simulink model "SIQBSC9LI"  (R2016a)
settings: Solver=VariableStepAuto  StartTime=0.0  StopTime=4/50  MaxStep=1e-6  MinStep=1e-7  RelTol=1e-3
libraries: powerlib x27
settings Model: Creator=satheeshwaran  LastModifiedBy=satheeshwaran

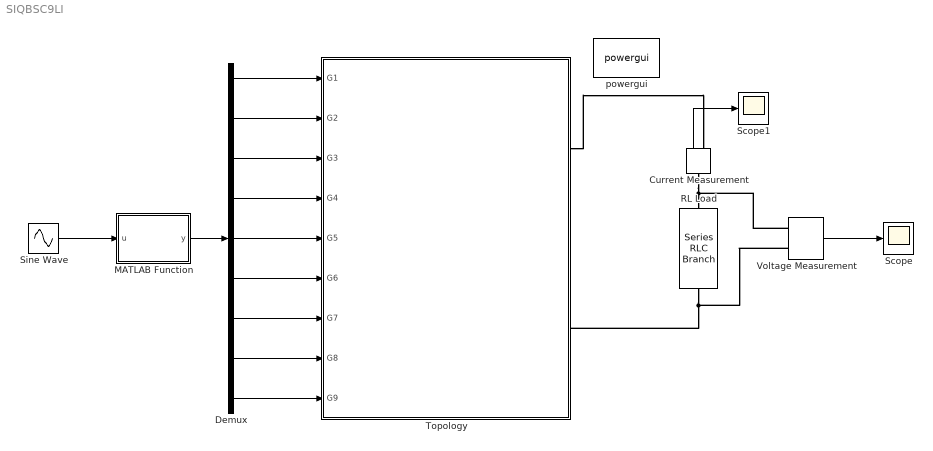
== system SIQBSC9LI ==
  Current Measurement : powerlib/Measurements/Current Measurement  PhasorSimulation=off  OutputType=Complex  PSBequivalent=0
  Demux : Demux  Outputs=9
  MATLAB Function : MATLAB Function  TreatAsAtomicUnit=on
  RL Load : powerlib/Elements/Series RLC Branch  LConnTagsString=__new0  RConnTagsString=__new0  BranchType=RL  Resistance=50  Inductance=0.1  SetiL0=off  InitialCurrent=0  Capacitance=1e-6  Setx0=off  InitialVoltage=0  Measurements=None
  Scope : Scope
  Scope1 : Scope
  Sine Wave : Sin  Amplitude=4  Frequency=2*pi*50  SampleTime=0
  Topology : Subsystem
  Voltage Measurement : powerlib/Measurements/Voltage Measurement  PhasorSimulation=off  OutputType=Complex  PSBequivalent=0
  powergui : powerlib/powergui  Priority=1  SimulationMode=Continuous  SolverType=Tustin/Backward Euler (TBE)  SampleTime=5e-6  frequency=60  SPID=off  DisableSnubberDevices=off  DisableRonSwitches=off  DisableVfSwitches=off  SwTol=0  DisplayEquations=off  Interpol=off  ExternalGateDelay=off  methode=off  Ts=10  FunctionMessages=off  echomessages=off  HookPort=off  EnableUseOfTLC=off  x0status=blocks  frequencyindice=0  Pbase=100e6  ErrMax=1e-4  Iterations=50  UnitsV=kV  UnitsW=MW  buscounter=0  RestoreLinks=warning  ResistiveCurrentMeasurement=off  Frange=[0:2:500]  Ylog=off  Xlog=on  ShowGrid=off  save=off  variable=ZData  structure=load  ZoomFFT=off  StartTime=0.08  cycles=1  DisplayStyle=1  fundamental=50  FreqAxis=off  MaxFrequency=10000  frequencyindicesteady=1  RmsSteady=1  display=off
  wires:
  Voltage Measurement/1 -> Scope/1
  Sine Wave/1 -> MATLAB Function/1(u)
  Demux/1 -> Topology/1(G1)
  Demux/2 -> Topology/2(G2)
  Demux/3 -> Topology/3(G3)
  Demux/4 -> Topology/4(G4)
  Demux/5 -> Topology/5(G5)
  Demux/6 -> Topology/6(G6)
  Demux/7 -> Topology/7(G7)
  Demux/8 -> Topology/8(G8)
  Demux/9 -> Topology/9(G9)
  MATLAB Function/1(y) -> Demux/1
  Current Measurement/1 -> Scope1/1
  connections:
  Voltage Measurement/LConn1 -- Current Measurement/LConn1 -- RL Load/LConn1
  RL Load/RConn1 -- Voltage Measurement/LConn2 -- Topology/RConn2
  Topology/RConn1 -- Current Measurement/RConn1

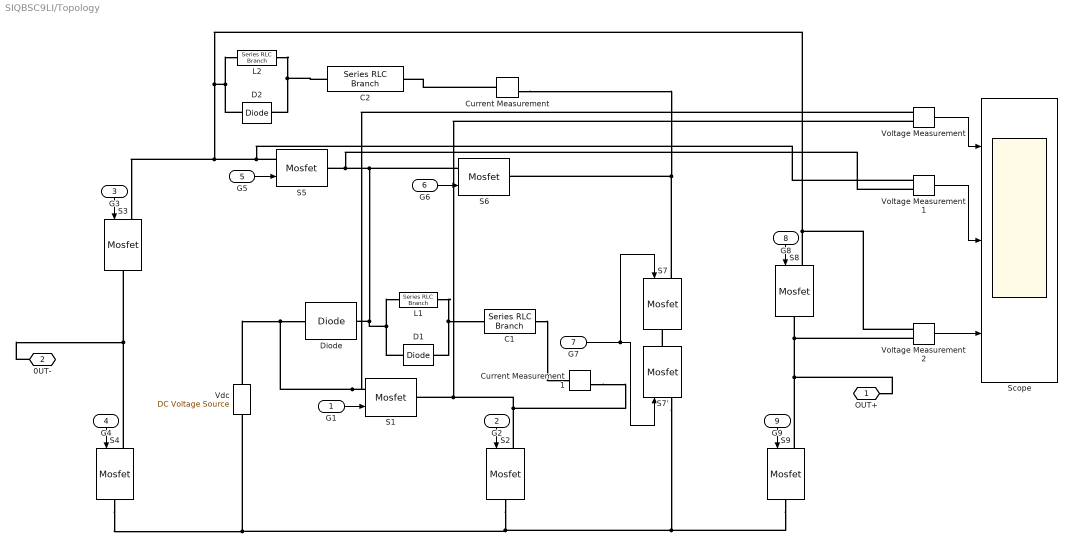
== system SIQBSC9LI/Topology ==
  G1 : Inport
  G2 : Inport  Port=2
  G3 : Inport  Port=3
  G4 : Inport  Port=4
  G5 : Inport  Port=5
  G6 : Inport  Port=6
  G7 : Inport  Port=7
  G8 : Inport  Port=8
  G9 : Inport  Port=9
  C1 : powerlib/Elements/Series RLC Branch  LConnTagsString=__new0  RConnTagsString=__new0  BranchType=C  Resistance=1  Inductance=1e-3  SetiL0=off  InitialCurrent=0  Capacitance=0.0033  Setx0=off  InitialVoltage=0  Measurements=None
  C2 : powerlib/Elements/Series RLC Branch  LConnTagsString=__new0  RConnTagsString=__new0  BranchType=C  Resistance=1  Inductance=1e-3  SetiL0=off  InitialCurrent=0  Capacitance=0.0032  Setx0=off  InitialVoltage=0  Measurements=None
  Current Measurement : powerlib/Measurements/Current Measurement  PhasorSimulation=off  OutputType=Complex  PSBequivalent=0
  Current Measurement1 : powerlib/Measurements/Current Measurement  PhasorSimulation=off  OutputType=Complex  PSBequivalent=0
  D1 : powerlib/Power Electronics/Diode  Ron=0.001  Lon=0  Vf=0  IC=0  UseSnubber=off  Rs=500  Cs=250e-9  Measurements=off
  D2 : powerlib/Power Electronics/Diode  Ron=0.001  Lon=0  Vf=0  IC=0  UseSnubber=off  Rs=500  Cs=250e-9  Measurements=off
  Diode : powerlib/Power Electronics/Diode  Ron=0.001  Lon=0  Vf=0  IC=0  UseSnubber=off  Rs=500  Cs=250e-9  Measurements=off
  L1 : powerlib/Elements/Series RLC Branch  LConnTagsString=__new0  RConnTagsString=__new0  BranchType=L  Resistance=1  Inductance=0.000011  SetiL0=off  InitialCurrent=0  Capacitance=1e-6  Setx0=off  InitialVoltage=0  Measurements=None
  L2 : powerlib/Elements/Series RLC Branch  LConnTagsString=__new0  RConnTagsString=__new0  BranchType=L  Resistance=1  Inductance=0.000048  SetiL0=off  InitialCurrent=0  Capacitance=1e-6  Setx0=off  InitialVoltage=0  Measurements=None
  S{1..9} (9 alike) : powerlib/Power Electronics/Mosfet  Ron=0.1  Lon=0  Rd=0.01  Vfd=0  IC=0  Rs=1e5  Cs=inf  Measurements=off
  S7' : powerlib/Power Electronics/Mosfet  Ron=0.1  Lon=0  Rd=0.01  Vfd=0  IC=0  Rs=1e5  Cs=inf  Measurements=off
  Scope : Scope  NumInputPorts=3
  Vdc : powerlib/Electrical Sources/DC Voltage Source  Amplitude=82  Measurements=None
  Voltage Measurement : powerlib/Measurements/Voltage Measurement  PhasorSimulation=off  OutputType=Complex  PSBequivalent=0
  Voltage Measurement1 : powerlib/Measurements/Voltage Measurement  PhasorSimulation=off  OutputType=Complex  PSBequivalent=0
  Voltage Measurement2 : powerlib/Measurements/Voltage Measurement  PhasorSimulation=off  OutputType=Complex  PSBequivalent=0
  OUT+ : PMIOPort  Port=1  Side=Right
  0UT- : PMIOPort  Port=2  Side=Right
  wires:
  G7/1 -> S7'/1, S7/1
  G3/1 -> S3/1
  G6/1 -> S6/1
  G8/1 -> S8/1
  G5/1 -> S5/1
  G1/1 -> S1/1
  G4/1 -> S4/1
  G2/1 -> S2/1
  G9/1 -> S9/1
  Voltage Measurement/1 -> Scope/1
  Voltage Measurement1/1 -> Scope/2
  Voltage Measurement2/1 -> Scope/3
  connections:
  S7'/RConn1 -- S7/RConn1
  S4/LConn1 -- 0UT-/RConn1 -- S3/RConn1
  D2/RConn1 -- Voltage Measurement2/LConn1 -- S8/LConn1 -- Voltage Measurement1/LConn1 -- S5/LConn1 -- S3/LConn1 -- L2/LConn1
  S2/RConn1 -- Vdc/LConn1 -- S4/RConn1 -- S7'/LConn1 -- S9/RConn1
  C1/RConn1 -- Current Measurement1/LConn1
  Current Measurement/LConn1 -- C2/RConn1
  S1/LConn1 -- Diode/LConn1 -- Vdc/RConn1 -- Voltage Measurement/LConn1
  S9/LConn1 -- OUT+/RConn1 -- S8/RConn1 -- Voltage Measurement2/LConn2
  C2/LConn1 -- D2/LConn1 -- L2/RConn1
  L1/RConn1 -- C1/LConn1 -- D1/LConn1
  S6/LConn1 -- Voltage Measurement1/LConn2 -- S5/RConn1 -- L1/LConn1 -- D1/RConn1 -- Diode/RConn1
  S7/LConn1 -- Current Measurement/RConn1 -- S6/RConn1
  S2/LConn1 -- S1/RConn1 -- Voltage Measurement/LConn2 -- Current Measurement1/RConn1

== matlab function SIQBSC9LI/MATLAB Function ==
  data: u input; y output
function y = fcn(u)

sine = u(1);
m = abs(sine);

s1=0; s2=0; s3=0; s4=0;
s5=0; s6=0; s7=0; s8=0; s9=0;

if (m <= 0.5)

    s2=1; s4=1; s9=1;

elseif (m <= 1.5)

    if (sine > 0)
        s2=1; s4=1; s5=1; s8=1;
    else
        s2=1; s3=1; s5=1; s9=1;
    end

elseif (m <= 2.5)

    if (sine > 0)
        s1=1; s4=1; s5=1; s7=1; s8=1;
    else
        s1=1; s3=1; s5=1; s7=1; s9=1;
    end

elseif (m <= 3.5)

    if (sine > 0)
        s2=1; s4=1; s6=1; s8=1;
    else
        s2=1; s3=1; s6=1; s9=1;
    end

elseif (m <= 4)

    if (sine > 0)
        s1=1; s4=1; s6=1; s8=1;
    else
        s1=1; s3=1; s6=1; s9=1;
    end

end

y = [s1; s2; s3; s4; s5; s6; s7; s8; s9];

end
